simulink model "HERIC"  (R2019a)
settings: Solver=VariableStepAuto  StartTime=0.0  StopTime=0.2  RelTol=1e-3
libraries: powerlib x21, powerlib_meascontrol x2
settings Model: Creator=Dell  LastModifiedBy=Dell

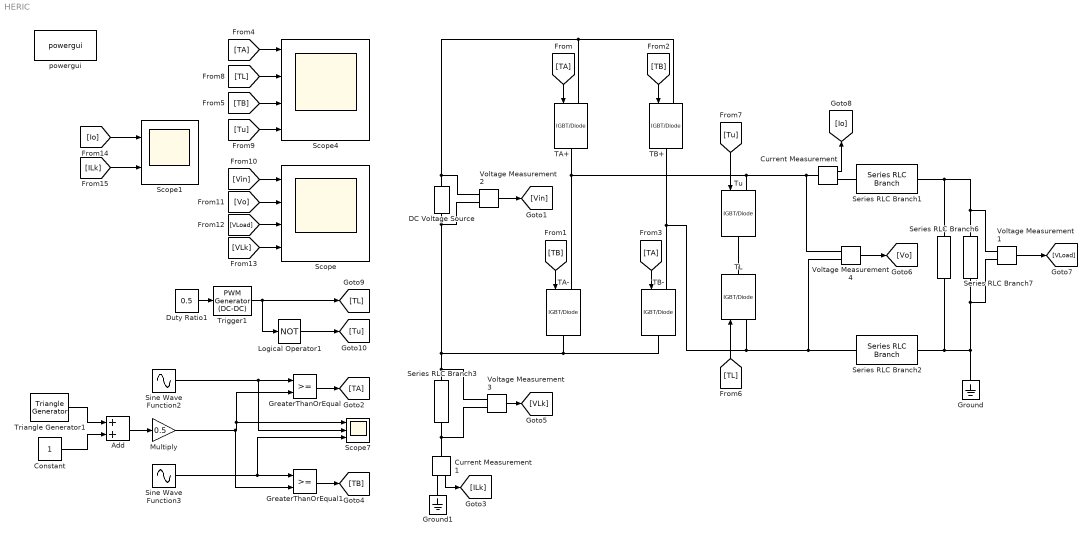
== system HERIC ==
  Add : Sum
  Constant : Constant
  Current Measurement : powerlib/Measurements/Current Measurement  PhasorSimulation=off  OutputType=Complex  PSBequivalent=0
      settings: SourceProductName=Simscape Electrical
  Current Measurement1 : powerlib/Measurements/Current Measurement  PhasorSimulation=off  OutputType=Complex  PSBequivalent=0
      settings: SourceProductName=Simscape Electrical
  DC Voltage Source : powerlib/Electrical Sources/DC Voltage Source  Amplitude=600  Measurements=None
      settings: SourceProductName=Simscape Electrical
  Duty Ratio1 : Constant  Value=0.5
  GreaterThanOrEqual : RelationalOperator  OutDataTypeStr=boolean  RndMeth=Simplest
  GreaterThanOrEqual1 : RelationalOperator  OutDataTypeStr=boolean  RndMeth=Simplest
  Ground : powerlib/Elements/Ground  LConnTagsString=a
      settings: SourceProductName=Simscape Electrical
  Ground1 : powerlib/Elements/Ground  LConnTagsString=a
      settings: SourceProductName=Simscape Electrical
  Logical Operator1 : Logic  Operator=NOT  AllPortsSameDT=off  OutDataTypeStr=boolean
  Multiply : Gain  Gain=0.5
  Scope : Scope  NumInputPorts=4
  Scope1 : Scope  NumInputPorts=2
  Scope4 : Scope  NumInputPorts=4
  Scope7 : Scope  NumInputPorts=3
  Series RLC Branch1 : powerlib/Elements/Series RLC Branch  LConnTagsString=__new0  RConnTagsString=__new0  BranchType=L  Resistance=1  Inductance=1e-03  SetiL0=off  InitialCurrent=0  Capacitance=1e-6  Setx0=off  InitialVoltage=0  Measurements=None
      settings: SourceProductName=Simscape Electrical
  Series RLC Branch2 : powerlib/Elements/Series RLC Branch  LConnTagsString=__new0  RConnTagsString=__new0  BranchType=L  Resistance=1  Inductance=1e-03  SetiL0=off  InitialCurrent=0  Capacitance=1e-6  Setx0=off  InitialVoltage=0  Measurements=None
      settings: SourceProductName=Simscape Electrical
  Series RLC Branch3 : powerlib/Elements/Series RLC Branch  LConnTagsString=__new0  RConnTagsString=__new0  BranchType=C  Resistance=1  Inductance=1e-3  SetiL0=off  InitialCurrent=0  Capacitance=100e-9  Setx0=off  InitialVoltage=0  Measurements=None
      settings: SourceProductName=Simscape Electrical
  Series RLC Branch6 : powerlib/Elements/Series RLC Branch  LConnTagsString=__new0  RConnTagsString=__new0  BranchType=C  Resistance=1  Inductance=1e-3  SetiL0=off  InitialCurrent=0  Capacitance=2e-6  Setx0=off  InitialVoltage=0  Measurements=None
      settings: SourceProductName=Simscape Electrical
  Series RLC Branch7 : powerlib/Elements/Series RLC Branch  LConnTagsString=__new0  RConnTagsString=__new0  BranchType=R  Resistance=10  Inductance=1e-3  SetiL0=off  InitialCurrent=0  Capacitance=1e-6  Setx0=off  InitialVoltage=0  Measurements=None
      settings: SourceProductName=Simscape Electrical
  Sine Wave Function2 : Sin  Amplitude=0.8  Frequency=2*pi*50.0  SampleTime=0
  Sine Wave Function3 : Sin  Amplitude=-0.8  Frequency=2*pi*50.0  SampleTime=0
  TA+ : powerlib/Power Electronics/IGBT//Diode  Ron=1e-3  Rs=1e5  Cs=inf  Measurements=off
      settings: SourceProductName=Simscape Electrical
  TA- : powerlib/Power Electronics/IGBT//Diode  Ron=1e-3  Rs=1e5  Cs=inf  Measurements=off
      settings: SourceProductName=Simscape Electrical
  TB+ : powerlib/Power Electronics/IGBT//Diode  Ron=1e-3  Rs=1e5  Cs=inf  Measurements=off
      settings: SourceProductName=Simscape Electrical
  TB- : powerlib/Power Electronics/IGBT//Diode  Ron=1e-3  Rs=1e5  Cs=inf  Measurements=off
      settings: SourceProductName=Simscape Electrical
  TL : powerlib/Power Electronics/IGBT//Diode  Ron=1e-3  Rs=1e5  Cs=inf  Measurements=off
      settings: SourceProductName=Simscape Electrical
  Triangle Generator1 : powerlib_meascontrol/Pulse & Signal Generators/Triangle Generator  Freq=10e3  Phase=0  Ts=1e-6
      settings: SourceProductName=Simscape Electrical
  Trigger1 : powerlib_meascontrol/Pulse & Signal Generators/PWM Generator (DC-DC)  Fsw=50  Ts=0
      settings: SourceProductName=Simscape Electrical
  Tu : powerlib/Power Electronics/IGBT//Diode  Ron=1e-3  Rs=1e5  Cs=inf  Measurements=off
      settings: SourceProductName=Simscape Electrical
  Voltage Measurement{1..4} (4 alike) : powerlib/Measurements/Voltage Measurement  PhasorSimulation=off  OutputType=Complex  PSBequivalent=0
      settings: SourceProductName=Simscape Electrical
  powergui : powerlib/powergui  Priority=1  SimulationMode=Discrete  SampleTime=1e-6  frequency=60  Iterations=50  frequencyindice=0  Pbase=100e6  ErrMax=1e-4  UnitsV=kV  UnitsW=MW  buscounter=0  FunctionMessages=off  echomessages=off  EnableUseOfTLC=off  CurrentSourceSwitches=off  DisableSnubberDevices=off  DisableRonSwitches=off  DisableVfSwitches=off  DisplayEquations=off  AutomaticDiscreteSolvers=off  SolverType=Tustin/Backward Euler (TBE)  Interpol=off  ExternalGateDelay=off  methode=off  Ts=100  x0status=blocks  SPID=on  SwTol=0  HookPort=off  NonlinearTolerance=0  nMaxIteration=15  ContinueOnMaxIteration=off  RestoreLinks=warning  ResistiveCurrentMeasurement=off  Frange=[0:2:500]  Ylog=off  Xlog=on  ShowGrid=off  save=off  variable=ZData  structure=0  ZoomFFT=off  StartTime=0.0  cycles=1  DisplayStyle=1  fundamental=60  FreqAxis=off  MaxFrequency=1000  frequencyindicesteady=1  RmsSteady=1  display=off
      settings: SourceProductName=Simscape Electrical
  wires:
  GreaterThanOrEqual/1 -> [TA]
  [TB] -> Scope4/3
  Current Measurement/1 -> [Io]
  Add/1 -> Multiply/1
  Triangle Generator1/1 -> Add/1
  Sine Wave Function3/1 -> GreaterThanOrEqual1/1, Scope7/3
  [TA] -> TB-/1
  Sine Wave Function2/1 -> Scope7/2, GreaterThanOrEqual/1
  [TB] -> TB+/1
  [TA] -> TA+/1
  GreaterThanOrEqual1/1 -> [TB]
  [VLoad] -> Scope/3
  [TA] -> Scope4/1
  Constant/1 -> Add/2
  Voltage Measurement3/1 -> [VLk]
  [TL] -> TL/1
  Trigger1/1 -> Logical Operator1/1, [TL]
  Voltage Measurement2/1 -> [Vin]
  [VLk] -> Scope/4
  Multiply/1 -> Scope7/1, GreaterThanOrEqual/2, GreaterThanOrEqual1/2
  Current Measurement1/1 -> [ILk]
  Logical Operator1/1 -> [Tu]
  [Vo] -> Scope/2
  Voltage Measurement1/1 -> [VLoad]
  [Tu] -> Tu/1
  [ILk] -> Scope1/2
  [TL] -> Scope4/2
  [Vin] -> Scope/1
  [Io] -> Scope1/1
  [Tu] -> Scope4/4
  Duty Ratio1/1 -> Trigger1/1
  Voltage Measurement4/1 -> [Vo]
  [TB] -> TA-/1
  connections:
  Current Measurement1/LConn1 -- Voltage Measurement3/LConn2 -- Series RLC Branch3/RConn1
  TB-/RConn1 -- TA-/RConn1 -- Series RLC Branch3/LConn1 -- Voltage Measurement3/LConn1 -- DC Voltage Source/LConn1 -- Voltage Measurement2/LConn2
  TA+/LConn1 -- DC Voltage Source/RConn1 -- Voltage Measurement2/LConn1 -- TB+/LConn1
  TA+/RConn1 -- Voltage Measurement4/LConn1 -- Current Measurement/LConn1 -- Tu/LConn1 -- TA-/LConn1
  Series RLC Branch2/LConn1 -- Series RLC Branch6/RConn1 -- Series RLC Branch7/RConn1 -- Voltage Measurement1/LConn2 -- Ground/LConn1
  Series RLC Branch1/RConn1 -- Series RLC Branch7/LConn1 -- Voltage Measurement1/LConn1 -- Series RLC Branch6/LConn1
  TL/LConn1 -- TB-/LConn1 -- TB+/RConn1 -- Series RLC Branch2/RConn1 -- Voltage Measurement4/LConn2
  TL/RConn1 -- Tu/RConn1
  Ground1/LConn1 -- Current Measurement1/RConn1
  Current Measurement/RConn1 -- Series RLC Branch1/LConn1
